simulink model "Demo_TollSystem_cs"  (R2014b)
settings: Solver=FixedStepDiscrete  StartTime=0.0  StopTime=13  FixedStep=1/20  RelTol=1e-3
PreLoadFcn:
  | mbxruntime.callbacks.PreLoadFcn(bdroot);
  | check_NUTS_defined
  | model_closed = 0;
  | assignin('base',['model_closed_' bdroot],false);
PostLoadFcn:
  | mbxruntime.callbacks.PostLoadFcn(bdroot);
InitFcn:
  | mbxruntime.callbacks.InitFcn(bdroot);
StartFcn:
  | mbxruntime.callbacks.StartFcn(bdroot);
  | 
  | open_system([bdroot '/Scope Plot']);
StopFcn:
  | mbxruntime.callbacks.StopFcn(bdroot);
model workspace: external: MAT-File .\Demo_TollSystem_cs_hws.mat (data not in the file)
undefined symbols (not defined in the file): Demo_TollSystem_cs_acfd828c7254e63e, Demo_TollSystem_cs_Mazda_RX8_1_Path_pathUniqueID
libraries: simulink x8, PreScanUsefulBlocks x4
(part 2 of 3)

== system Demo_TollSystem_cs/RFBeacon_3 ==
  Sensor : S-Function  FunctionName=sfun_Beacon  Parameters=sensorID, NrEntitiesOut, timestep  EnableBusSupport=off  mask(PreScan Source Block: RFBeacon I/O){sensorID=44, NrEntitiesOut=5, timestep=1/20}
      mask prompts: sensorID "Sensor ID"; NrEntitiesOut "User Specified: # of Visible OBUs"; timestep "MATLAB timestep:"
      mask help:
      | Using the Beacon and OBU (On-Board Unit) information between actors and infrastructure can be exchanged.
      |
      | The Beacon Receiver receives actor information and user-definable signals.
      |
      | For more information, please click Help.
      mask Help: eval('openHelp(486)')
      mask Display: image(imread('ico_Beacon_RF_24_gray.png'))
  RFBeacon_3 : Outport  Tag=outport/BeaconAndOBU/RFBeaconSensor  OutDataTypeStr=Bus: PRESCAN_BEACON_MESSAGE  PortDimensions=5  SampleTime=1/20
  wires:
  Sensor/1 -> RFBeacon_3/1

== system Demo_TollSystem_cs/RFBeacon_3Out ==
  RFBeacon_3Out : Inport  Tag=inport/BeaconAndOBU/RFBeaconSensor  OutDataTypeStr=Bus: PRESCAN_BEACONOBU_INPUT_DATA  PortDimensions=1  SampleTime=1/20  BusOutputAsStruct=on
  Actuator : S-Function  FunctionName=sfun_BeaconOBU_Input  Parameters=sensorID, timestep  EnableBusSupport=off  mask(PreScan Sink Block: RFBeacon I/O){sensorID=44, timestep=1/20}
      mask prompts: sensorID "Sensor ID"; timestep "MATLAB timestep:"
      mask help:
      | Using the Beacon and OBU (On-Board Unit) information between actors and infrastructure can be exchanged.
      |
      | The Beacon Transmitter contains the following, user-definable signals:
      |
      | - Beacon Type		[-]
      | - Spares (1:15)		[-]
      |
      | For more information, please click Help.
      mask Help: eval('openHelp(486)')
      mask Display: image(imread('ico_Beacon_RF_24_gray.png'))
  wires:
  RFBeacon_3Out/1 -> Actuator/1

== system Demo_TollSystem_cs/RFOBU_1 ==
  Sensor : S-Function  FunctionName=sfun_OBU  Parameters=sensorID, NrEntitiesOut, timestep  EnableBusSupport=off  mask(PreScan Source Block: RFOBU I/O){sensorID=17, NrEntitiesOut=2, timestep=1/20}
      mask prompts: sensorID "Sensor ID"; NrEntitiesOut "User Specified: # of Visible OBUs"; timestep "MATLAB timestep:"
      mask help:
      | Using the Beacon and OBU (On-Board Unit) information between actors and infrastructure can be exchanged.
      |
      | The OBU Receiver receives infrastructure information and user-definable signals.
      |
      | For more information, please click Help.
      mask Help: eval('openHelp(487)')
      mask Display: image(imread('ico_OBU_RF_24_gray.png'))
  RFOBU_1 : Outport  Tag=outport/BeaconAndOBU/RFOBU  OutDataTypeStr=Bus: PRESCAN_OBU_MESSAGE  PortDimensions=2  SampleTime=1/20
  wires:
  Sensor/1 -> RFOBU_1/1

== system Demo_TollSystem_cs/RFOBU_1Out ==
  RFOBU_1Out : Inport  Tag=inport/BeaconAndOBU/RFOBU  OutDataTypeStr=Bus: PRESCAN_BEACONOBU_INPUT_DATA  PortDimensions=1  SampleTime=1/20  BusOutputAsStruct=on
  Actuator : S-Function  FunctionName=sfun_BeaconOBU_Input  Parameters=sensorID, timestep  EnableBusSupport=off  mask(PreScan Sink Block: RFOBU I/O){sensorID=17, timestep=1/20}
      mask prompts: sensorID "Sensor ID"; timestep "MATLAB timestep:"
      mask help:
      | Using the Beacon and OBU (On-Board Unit) information between actors and infrastructure can be exchanged.
      |
      | The OBU Transmitter contains the following, user-definable signals:
      |
      | - Vehicle Type		[-]
      | - Spares (1:15)		[-]
      |
      | For more information, please click Help.
      mask Help: eval('openHelp(487)')
      mask Display: image(imread('ico_OBU_RF_24_gray.png'))
  wires:
  RFOBU_1Out/1 -> Actuator/1

== system Demo_TollSystem_cs/SELF_Mazda_RX8_1 ==
  Sensor : S-Function  FunctionName=sfun_SelfSensor  Parameters=UniqueID, TimeStep  EnableBusSupport=off  mask(PreScan Source Block: SELF){UniqueID=16, TimeStep=1/20}
      mask prompts: UniqueID "Auto-Assigned: Unique ID"; TimeStep "Auto-Assigned: Upload Period [s]"
      mask help:
      | The SELF port shows (state) information of the actor itself. The outputs are position in the experiment's axis system and the GPS coordinates, and the object's absolute velocity and compass heading.
      |
      | For more information, please click Help.
      mask Help: eval('openHelp(462)')
      mask Display: image(imread('GPS.png'))
  SELF_Mazda_RX8_1 : Outport  Tag=outport/SelfPort  OutDataTypeStr=Bus: PRESCAN_SELFSENSORDATA  PortDimensions=1  SampleTime=1/20
  wires:
  Sensor/1 -> SELF_Mazda_RX8_1/1

== system Demo_TollSystem_cs/STATE_Mazda_RX8_1_bus ==
  STATE_Mazda_RX8_1_bus : Inport  Tag=inport/StatePort  OutDataTypeStr=Bus: PRESCAN_STATEACTUATORDATA  PortDimensions=1  SampleTime=1/20  BusOutputAsStruct=on
  Actuator : S-Function  FunctionName=sfun_StateActuator  Parameters=UniqueID, TimeStep  EnableBusSupport=off  mask(PreScan Sink Block: State){UniqueID=16, TimeStep=1/20}
      mask prompts: UniqueID "Auto-Assigned: Unique ID"; TimeStep "Auto-Assigned: Upload Period [s]"
      mask help:
      | The Actor State contains a vector signal of size (9x1), containing the following signals:
      |
      | -  Position    	(x,y,z)             	[m]
      | -  Velocity    	(vx,vy,vz)         	[m/s]
      | -  Angles       	(Roll, Pitch, Yaw)	[rad]
      |
      | The Actor state is defined in the global axis system.
      | The state is superponed on the Initial position defined in the GUI.
      |
      | For more information, please click Help.
      mask Help: eval('openHelp(222)')
      mask Display: image(imread('State.png'))
  wires:
  STATE_Mazda_RX8_1_bus/1 -> Actuator/1

== system Demo_TollSystem_cs/ScenarioEngine ==
  Clock : Clock
  sfun_ScenarioEngine : S-Function  FunctionName=sfun_ScenarioEngine  Parameters=TimeStep  EnableBusSupport=off
  wires:
  Clock/1 -> sfun_ScenarioEngine/1

== system Demo_TollSystem_cs/Synchronizer ==
  Bus Selector1 : BusSelector  OutputSignals=FederateStopped
  Stop Simulation : Stop
  sfun_Synchronizer : S-Function  FunctionName=sfun_Synchronizer  Parameters=SampleTime  EnableBusSupport=off  mask(Legacy Function){SFunctionSpec=void prescan_synchronizer_outputFcn(void ** work1, PRESCAN_SYNCHRONIZEDATA y1[1]), SampleTime=TimeStep, ShowSpec=on}
      mask prompts: SampleTime "Sample time (-1 for inherited):"; ShowSpec "Display function specification"
      mask help:
      | This block allows you to call the legacy functions specified by the following Legacy Code Tool definition:
      | def.SFunctionName = 'sfun_Synchronizer';
      | def.OutputFcnSpec = 'void prescan_synchronizer_outputFcn(void ** work1, PRESCAN_SYNCHRONIZEDATA y1[1])';
      | def.StartFcnSpec = 'void prescan_synchronizer_startFcn(void ** work1)';
      | def.TerminateFcnSpec = 'void prescan_synchronizer_terminateFcn(void ** work1)';
      | def.HeaderFiles = {'prescan_synchronizer_data.h'};
      | def.HostLibFiles = {'sensorinterfaced.lib'};
      | def.IncPaths = {'src', 'C:\prescandev\vislibrary\vis\..\pimp\include\sensors\InterfaceRTW'};
      | def.SrcPaths = {'src'};
      | def.LibPaths = {'C:\\prescandev\\vislibrary_build\lib'};
      | def.SampleTime = 'parameterized';
      | def.Options.language = 'C';
      mask Help: <p>This block was generated automatically by the Legacy Code Tool. For detailed help on this tool, call<a href="matlab:legacy_code('help')"> legacy_code('help')</a>.</p>
      mask Callback ShowSpec:
      | if strcmp(get_param(gcbh, 'ShowSpec'), 'on')
      |   set_param(gcbh, 'MaskDisplay', sprintf('fprintf(''%s'');', get_param(gcbh, 'SFunctionSpec')));
      | else
      |   set_param(gcbh, 'MaskDisplay', sprintf('fprintf(''%s'');', get_param(gcbh, 'FunctionName')));
      | end
      mask Display: fprintf('void prescan_synchronizer_outputFcn(void ** work1, PRESCAN_SYNCHRONIZEDATA y1[1])');
  wires:
  Bus Selector1/1 -> Stop Simulation/1  "<FederateStopped>"
  sfun_Synchronizer/1 -> Bus Selector1/1

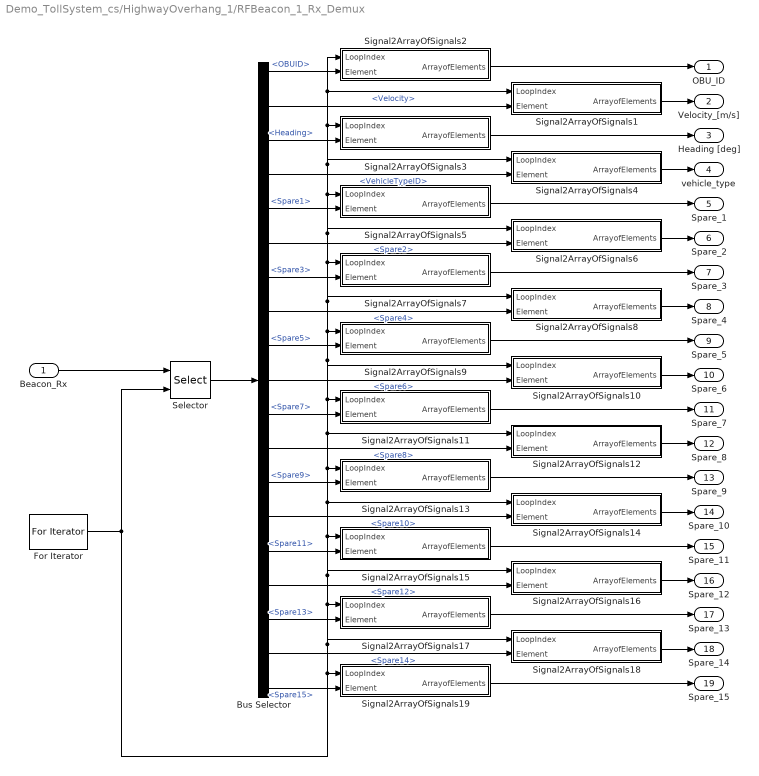
== system Demo_TollSystem_cs/HighwayOverhang_1/RFBeacon_1_Rx_Demux ==
  Beacon_Rx : Inport
  Bus Selector : BusSelector  OutputSignals=DATA.OBUID,DATA.Velocity,DATA.Heading,DATA.VehicleTypeID,DATA.Spare1,DATA.Spare2,DATA.Spare3,DATA.Spare4,DATA.Spare5,DATA.Spare6,DATA.Spare7,DATA.Spare8,DATA.Spare9,DATA.Spare10,DATA.Spare11,DATA.Spare12,DATA.Spare13,DATA.Spare14,DATA.Spare15
  For Iterator : ForIterator  ResetStates=reset  IterationLimit=detectableObjects
  Selector : Selector  InputPortWidth=detectableObjects  IndexOptions=Index vector (port)  Indices=[1 3]
  Signal2ArrayOfSignals1 : Subsystem  mask{VECTORLENGTH=detectableObjects}
      mask prompts: VECTORLENGTH "Length of vector"
  Signal2ArrayOfSignals10 : Subsystem  mask{VECTORLENGTH=detectableObjects}
      mask prompts: VECTORLENGTH "Length of vector"
  Signal2ArrayOfSignals11 : Subsystem  mask{VECTORLENGTH=detectableObjects}
      mask prompts: VECTORLENGTH "Length of vector"
  Signal2ArrayOfSignals12 : Subsystem  mask{VECTORLENGTH=detectableObjects}
      mask prompts: VECTORLENGTH "Length of vector"
  Signal2ArrayOfSignals13 : Subsystem  mask{VECTORLENGTH=detectableObjects}
      mask prompts: VECTORLENGTH "Length of vector"
  Signal2ArrayOfSignals14 : Subsystem  mask{VECTORLENGTH=detectableObjects}
      mask prompts: VECTORLENGTH "Length of vector"
  Signal2ArrayOfSignals15 : Subsystem  mask{VECTORLENGTH=detectableObjects}
      mask prompts: VECTORLENGTH "Length of vector"
  Signal2ArrayOfSignals16 : Subsystem  mask{VECTORLENGTH=detectableObjects}
      mask prompts: VECTORLENGTH "Length of vector"
  Signal2ArrayOfSignals17 : Subsystem  mask{VECTORLENGTH=detectableObjects}
      mask prompts: VECTORLENGTH "Length of vector"
  Signal2ArrayOfSignals18 : Subsystem  mask{VECTORLENGTH=detectableObjects}
      mask prompts: VECTORLENGTH "Length of vector"
  Signal2ArrayOfSignals19 : Subsystem  mask{VECTORLENGTH=detectableObjects}
      mask prompts: VECTORLENGTH "Length of vector"
  Signal2ArrayOfSignals2 : Subsystem  mask{VECTORLENGTH=detectableObjects}
      mask prompts: VECTORLENGTH "Length of vector"
  Signal2ArrayOfSignals3 : Subsystem  mask{VECTORLENGTH=detectableObjects}
      mask prompts: VECTORLENGTH "Length of vector"
  Signal2ArrayOfSignals4 : Subsystem  mask{VECTORLENGTH=detectableObjects}
      mask prompts: VECTORLENGTH "Length of vector"
  Signal2ArrayOfSignals5 : Subsystem  mask{VECTORLENGTH=detectableObjects}
      mask prompts: VECTORLENGTH "Length of vector"
  Signal2ArrayOfSignals6 : Subsystem  mask{VECTORLENGTH=detectableObjects}
      mask prompts: VECTORLENGTH "Length of vector"
  Signal2ArrayOfSignals7 : Subsystem  mask{VECTORLENGTH=detectableObjects}
      mask prompts: VECTORLENGTH "Length of vector"
  Signal2ArrayOfSignals8 : Subsystem  mask{VECTORLENGTH=detectableObjects}
      mask prompts: VECTORLENGTH "Length of vector"
  Signal2ArrayOfSignals9 : Subsystem  mask{VECTORLENGTH=detectableObjects}
      mask prompts: VECTORLENGTH "Length of vector"
  OBU_ID : Outport
  Velocity_[m/s] : Outport  Port=2
  Heading [deg] : Outport  Port=3
  vehicle_type : Outport  Port=4
  Spare_1 : Outport  Port=5
  Spare_2 : Outport  Port=6
  Spare_3 : Outport  Port=7
  Spare_4 : Outport  Port=8
  Spare_5 : Outport  Port=9
  Spare_6 : Outport  Port=10
  Spare_7 : Outport  Port=11
  Spare_8 : Outport  Port=12
  Spare_9 : Outport  Port=13
  Spare_10 : Outport  Port=14
  Spare_11 : Outport  Port=15
  Spare_12 : Outport  Port=16
  Spare_13 : Outport  Port=17
  Spare_14 : Outport  Port=18
  Spare_15 : Outport  Port=19
  wires:
  Beacon_Rx/1 -> Selector/1
  For Iterator/1 -> Selector/2, Signal2ArrayOfSignals19/1(LoopIndex), Signal2ArrayOfSignals17/1(LoopIndex), Signal2ArrayOfSignals15/1(LoopIndex), Signal2ArrayOfSignals13/1(LoopIndex), Signal2ArrayOfSignals11/1(LoopIndex), Signal2ArrayOfSignals9/1(LoopIndex), Signal2ArrayOfSignals7/1(LoopIndex), Signal2ArrayOfSignals5/1(LoopIndex), Signal2ArrayOfSignals3/1(LoopIndex), Signal2ArrayOfSignals2/1(LoopIndex), Signal2ArrayOfSignals1/1(LoopIndex), Signal2ArrayOfSignals4/1(LoopIndex), Signal2ArrayOfSignals6/1(LoopIndex), Signal2ArrayOfSignals8/1(LoopIndex), Signal2ArrayOfSignals10/1(LoopIndex), Signal2ArrayOfSignals12/1(LoopIndex), Signal2ArrayOfSignals14/1(LoopIndex), Signal2ArrayOfSignals16/1(LoopIndex), Signal2ArrayOfSignals18/1(LoopIndex)
  Selector/1 -> Bus Selector/1
  Bus Selector/1 -> Signal2ArrayOfSignals2/2(Element)  "<OBUID>"
  Signal2ArrayOfSignals2/1(ArrayofElements) -> OBU_ID/1
  Bus Selector/2 -> Signal2ArrayOfSignals1/2(Element)  "<Velocity>"
  Signal2ArrayOfSignals1/1(ArrayofElements) -> Velocity_[m/s]/1
  Bus Selector/3 -> Signal2ArrayOfSignals3/2(Element)  "<Heading>"
  Signal2ArrayOfSignals3/1(ArrayofElements) -> Heading [deg]/1
  Bus Selector/4 -> Signal2ArrayOfSignals4/2(Element)  "<VehicleTypeID>"
  Signal2ArrayOfSignals4/1(ArrayofElements) -> vehicle_type/1
  Bus Selector/5 -> Signal2ArrayOfSignals5/2(Element)  "<Spare1>"
  Signal2ArrayOfSignals5/1(ArrayofElements) -> Spare_1/1
  Bus Selector/6 -> Signal2ArrayOfSignals6/2(Element)  "<Spare2>"
  Signal2ArrayOfSignals6/1(ArrayofElements) -> Spare_2/1
  Bus Selector/7 -> Signal2ArrayOfSignals7/2(Element)  "<Spare3>"
  Signal2ArrayOfSignals7/1(ArrayofElements) -> Spare_3/1
  Bus Selector/8 -> Signal2ArrayOfSignals8/2(Element)  "<Spare4>"
  Signal2ArrayOfSignals8/1(ArrayofElements) -> Spare_4/1
  Bus Selector/9 -> Signal2ArrayOfSignals9/2(Element)  "<Spare5>"
  Bus Selector/10 -> Signal2ArrayOfSignals10/2(Element)  "<Spare6>"
  Bus Selector/11 -> Signal2ArrayOfSignals11/2(Element)  "<Spare7>"
  Bus Selector/12 -> Signal2ArrayOfSignals12/2(Element)  "<Spare8>"
  Signal2ArrayOfSignals9/1(ArrayofElements) -> Spare_5/1
  Signal2ArrayOfSignals10/1(ArrayofElements) -> Spare_6/1
  Signal2ArrayOfSignals11/1(ArrayofElements) -> Spare_7/1
  Signal2ArrayOfSignals12/1(ArrayofElements) -> Spare_8/1
  Bus Selector/13 -> Signal2ArrayOfSignals13/2(Element)  "<Spare9>"
  Bus Selector/14 -> Signal2ArrayOfSignals14/2(Element)  "<Spare10>"
  Signal2ArrayOfSignals13/1(ArrayofElements) -> Spare_9/1
  Signal2ArrayOfSignals14/1(ArrayofElements) -> Spare_10/1
  Bus Selector/15 -> Signal2ArrayOfSignals15/2(Element)  "<Spare11>"
  Signal2ArrayOfSignals15/1(ArrayofElements) -> Spare_11/1
  Bus Selector/16 -> Signal2ArrayOfSignals16/2(Element)  "<Spare12>"
  Signal2ArrayOfSignals16/1(ArrayofElements) -> Spare_12/1
  Bus Selector/17 -> Signal2ArrayOfSignals17/2(Element)  "<Spare13>"
  Signal2ArrayOfSignals17/1(ArrayofElements) -> Spare_13/1
  Bus Selector/18 -> Signal2ArrayOfSignals18/2(Element)  "<Spare14>"
  Signal2ArrayOfSignals18/1(ArrayofElements) -> Spare_14/1
  Bus Selector/19 -> Signal2ArrayOfSignals19/2(Element)  "<Spare15>"
  Signal2ArrayOfSignals19/1(ArrayofElements) -> Spare_15/1

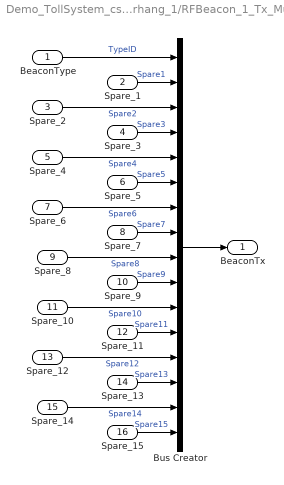
== system Demo_TollSystem_cs/HighwayOverhang_1/RFBeacon_1_Tx_Mux ==
  BeaconType : Inport
  Spare_1 : Inport  Port=2
  Spare_2 : Inport  Port=3
  Spare_3 : Inport  Port=4
  Spare_4 : Inport  Port=5
  Spare_5 : Inport  Port=6
  Spare_6 : Inport  Port=7
  Spare_7 : Inport  Port=8
  Spare_8 : Inport  Port=9
  Spare_9 : Inport  Port=10
  Spare_10 : Inport  Port=11
  Spare_11 : Inport  Port=12
  Spare_12 : Inport  Port=13
  Spare_13 : Inport  Port=14
  Spare_14 : Inport  Port=15
  Spare_15 : Inport  Port=16
  Bus Creator : BusCreator  Inputs=16  OutDataTypeStr=Bus: PRESCAN_BEACONOBU_INPUT_DATA
  BeaconTx : Outport
  wires:
  Spare_11/1 -> Bus Creator/12  "Spare11"
  Spare_12/1 -> Bus Creator/13  "Spare12"
  Spare_13/1 -> Bus Creator/14  "Spare13"
  Spare_14/1 -> Bus Creator/15  "Spare14"
  Spare_15/1 -> Bus Creator/16  "Spare15"
  Spare_1/1 -> Bus Creator/2  "Spare1"
  Spare_2/1 -> Bus Creator/3  "Spare2"
  Spare_3/1 -> Bus Creator/4  "Spare3"
  Spare_4/1 -> Bus Creator/5  "Spare4"
  Spare_5/1 -> Bus Creator/6  "Spare5"
  Spare_6/1 -> Bus Creator/7  "Spare6"
  Spare_7/1 -> Bus Creator/8  "Spare7"
  Spare_8/1 -> Bus Creator/9  "Spare8"
  Spare_9/1 -> Bus Creator/10  "Spare9"
  Spare_10/1 -> Bus Creator/11  "Spare10"
  Bus Creator/1 -> BeaconTx/1
  BeaconType/1 -> Bus Creator/1  "TypeID"

== system Demo_TollSystem_cs/HighwayOverhang_1/threshold check ==
  Lat : Inport
  Lon : Inport  Port=2
  Pos Lat : Inport  Port=3
  Pos Lon : Inport  Port=4
  Abs : Abs
  Abs1 : Abs
  Accuracy : Constant  Value=1e-5
  Compare To Zero : simulink/Logic and Bit Operations/Compare To Zero  relop=~=  OutDataTypeStr=uint8  ZeroCross=off
  Compare To Zero1 : simulink/Logic and Bit Operations/Compare To Zero  relop=~=  OutDataTypeStr=uint8  ZeroCross=off
  Logical Operator : Logic  Inputs=3  AllPortsSameDT=off  OutDataTypeStr=boolean
  Logical Operator1 : Logic  Operator=OR  AllPortsSameDT=off  OutDataTypeStr=boolean
  Relational Operator : RelationalOperator  Operator=>  OutDataTypeStr=boolean
  Relational Operator1 : RelationalOperator  Operator=>  OutDataTypeStr=boolean
  Sum : Sum  Inputs=|+-
  Sum1 : Sum  Inputs=|+-
  Out : Outport
  wires:
  Pos Lat/1 -> Sum/2
  Lat/1 -> Sum/1, Compare To Zero/1
  Sum/1 -> Abs/1
  Pos Lon/1 -> Sum1/2
  Lon/1 -> Sum1/1, Compare To Zero1/1
  Sum1/1 -> Abs1/1
  Relational Operator/1 -> Logical Operator1/1
  Logical Operator/1 -> Out/1
  Abs/1 -> Relational Operator/1
  Accuracy/1 -> Relational Operator/2, Relational Operator1/2
  Abs1/1 -> Relational Operator1/1
  Compare To Zero/1 -> Logical Operator/1
  Compare To Zero1/1 -> Logical Operator1/2
  Relational Operator1/1 -> Logical Operator/3
  Logical Operator1/1 -> Logical Operator/2

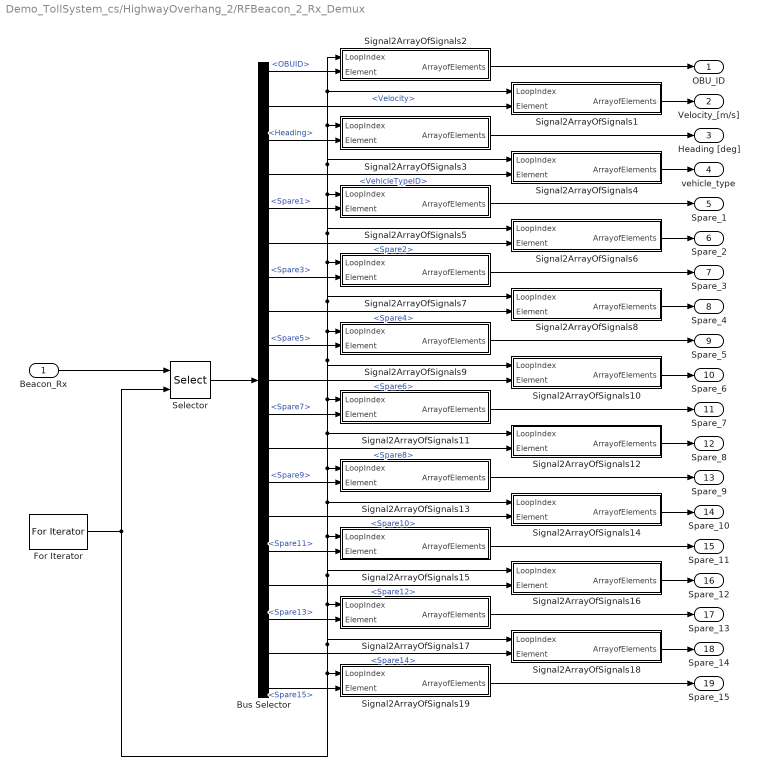
== system Demo_TollSystem_cs/HighwayOverhang_2/RFBeacon_2_Rx_Demux ==
  Beacon_Rx : Inport
  Bus Selector : BusSelector  OutputSignals=DATA.OBUID,DATA.Velocity,DATA.Heading,DATA.VehicleTypeID,DATA.Spare1,DATA.Spare2,DATA.Spare3,DATA.Spare4,DATA.Spare5,DATA.Spare6,DATA.Spare7,DATA.Spare8,DATA.Spare9,DATA.Spare10,DATA.Spare11,DATA.Spare12,DATA.Spare13,DATA.Spare14,DATA.Spare15
  For Iterator : ForIterator  ResetStates=reset  IterationLimit=detectableObjects
  Selector : Selector  InputPortWidth=detectableObjects  IndexOptions=Index vector (port)  Indices=[1 3]
  Signal2ArrayOfSignals1 : Subsystem  mask{VECTORLENGTH=detectableObjects}
      mask prompts: VECTORLENGTH "Length of vector"
  Signal2ArrayOfSignals10 : Subsystem  mask{VECTORLENGTH=detectableObjects}
      mask prompts: VECTORLENGTH "Length of vector"
  Signal2ArrayOfSignals11 : Subsystem  mask{VECTORLENGTH=detectableObjects}
      mask prompts: VECTORLENGTH "Length of vector"
  Signal2ArrayOfSignals12 : Subsystem  mask{VECTORLENGTH=detectableObjects}
      mask prompts: VECTORLENGTH "Length of vector"
  Signal2ArrayOfSignals13 : Subsystem  mask{VECTORLENGTH=detectableObjects}
      mask prompts: VECTORLENGTH "Length of vector"
  Signal2ArrayOfSignals14 : Subsystem  mask{VECTORLENGTH=detectableObjects}
      mask prompts: VECTORLENGTH "Length of vector"
  Signal2ArrayOfSignals15 : Subsystem  mask{VECTORLENGTH=detectableObjects}
      mask prompts: VECTORLENGTH "Length of vector"
  Signal2ArrayOfSignals16 : Subsystem  mask{VECTORLENGTH=detectableObjects}
      mask prompts: VECTORLENGTH "Length of vector"
  Signal2ArrayOfSignals17 : Subsystem  mask{VECTORLENGTH=detectableObjects}
      mask prompts: VECTORLENGTH "Length of vector"
  Signal2ArrayOfSignals18 : Subsystem  mask{VECTORLENGTH=detectableObjects}
      mask prompts: VECTORLENGTH "Length of vector"
  Signal2ArrayOfSignals19 : Subsystem  mask{VECTORLENGTH=detectableObjects}
      mask prompts: VECTORLENGTH "Length of vector"
  Signal2ArrayOfSignals2 : Subsystem  mask{VECTORLENGTH=detectableObjects}
      mask prompts: VECTORLENGTH "Length of vector"
  Signal2ArrayOfSignals3 : Subsystem  mask{VECTORLENGTH=detectableObjects}
      mask prompts: VECTORLENGTH "Length of vector"
  Signal2ArrayOfSignals4 : Subsystem  mask{VECTORLENGTH=detectableObjects}
      mask prompts: VECTORLENGTH "Length of vector"
  Signal2ArrayOfSignals5 : Subsystem  mask{VECTORLENGTH=detectableObjects}
      mask prompts: VECTORLENGTH "Length of vector"
  Signal2ArrayOfSignals6 : Subsystem  mask{VECTORLENGTH=detectableObjects}
      mask prompts: VECTORLENGTH "Length of vector"
  Signal2ArrayOfSignals7 : Subsystem  mask{VECTORLENGTH=detectableObjects}
      mask prompts: VECTORLENGTH "Length of vector"
  Signal2ArrayOfSignals8 : Subsystem  mask{VECTORLENGTH=detectableObjects}
      mask prompts: VECTORLENGTH "Length of vector"
  Signal2ArrayOfSignals9 : Subsystem  mask{VECTORLENGTH=detectableObjects}
      mask prompts: VECTORLENGTH "Length of vector"
  OBU_ID : Outport
  Velocity_[m/s] : Outport  Port=2
  Heading [deg] : Outport  Port=3
  vehicle_type : Outport  Port=4
  Spare_1 : Outport  Port=5
  Spare_2 : Outport  Port=6
  Spare_3 : Outport  Port=7
  Spare_4 : Outport  Port=8
  Spare_5 : Outport  Port=9
  Spare_6 : Outport  Port=10
  Spare_7 : Outport  Port=11
  Spare_8 : Outport  Port=12
  Spare_9 : Outport  Port=13
  Spare_10 : Outport  Port=14
  Spare_11 : Outport  Port=15
  Spare_12 : Outport  Port=16
  Spare_13 : Outport  Port=17
  Spare_14 : Outport  Port=18
  Spare_15 : Outport  Port=19
  wires:
  Beacon_Rx/1 -> Selector/1
  For Iterator/1 -> Selector/2, Signal2ArrayOfSignals19/1(LoopIndex), Signal2ArrayOfSignals17/1(LoopIndex), Signal2ArrayOfSignals15/1(LoopIndex), Signal2ArrayOfSignals13/1(LoopIndex), Signal2ArrayOfSignals11/1(LoopIndex), Signal2ArrayOfSignals9/1(LoopIndex), Signal2ArrayOfSignals7/1(LoopIndex), Signal2ArrayOfSignals5/1(LoopIndex), Signal2ArrayOfSignals3/1(LoopIndex), Signal2ArrayOfSignals2/1(LoopIndex), Signal2ArrayOfSignals1/1(LoopIndex), Signal2ArrayOfSignals4/1(LoopIndex), Signal2ArrayOfSignals6/1(LoopIndex), Signal2ArrayOfSignals8/1(LoopIndex), Signal2ArrayOfSignals10/1(LoopIndex), Signal2ArrayOfSignals12/1(LoopIndex), Signal2ArrayOfSignals14/1(LoopIndex), Signal2ArrayOfSignals16/1(LoopIndex), Signal2ArrayOfSignals18/1(LoopIndex)
  Selector/1 -> Bus Selector/1
  Bus Selector/1 -> Signal2ArrayOfSignals2/2(Element)  "<OBUID>"
  Signal2ArrayOfSignals2/1(ArrayofElements) -> OBU_ID/1
  Bus Selector/2 -> Signal2ArrayOfSignals1/2(Element)  "<Velocity>"
  Signal2ArrayOfSignals1/1(ArrayofElements) -> Velocity_[m/s]/1
  Bus Selector/3 -> Signal2ArrayOfSignals3/2(Element)  "<Heading>"
  Signal2ArrayOfSignals3/1(ArrayofElements) -> Heading [deg]/1
  Bus Selector/4 -> Signal2ArrayOfSignals4/2(Element)  "<VehicleTypeID>"
  Signal2ArrayOfSignals4/1(ArrayofElements) -> vehicle_type/1
  Bus Selector/5 -> Signal2ArrayOfSignals5/2(Element)  "<Spare1>"
  Signal2ArrayOfSignals5/1(ArrayofElements) -> Spare_1/1
  Bus Selector/6 -> Signal2ArrayOfSignals6/2(Element)  "<Spare2>"
  Signal2ArrayOfSignals6/1(ArrayofElements) -> Spare_2/1
  Bus Selector/7 -> Signal2ArrayOfSignals7/2(Element)  "<Spare3>"
  Signal2ArrayOfSignals7/1(ArrayofElements) -> Spare_3/1
  Bus Selector/8 -> Signal2ArrayOfSignals8/2(Element)  "<Spare4>"
  Signal2ArrayOfSignals8/1(ArrayofElements) -> Spare_4/1
  Bus Selector/9 -> Signal2ArrayOfSignals9/2(Element)  "<Spare5>"
  Bus Selector/10 -> Signal2ArrayOfSignals10/2(Element)  "<Spare6>"
  Bus Selector/11 -> Signal2ArrayOfSignals11/2(Element)  "<Spare7>"
  Bus Selector/12 -> Signal2ArrayOfSignals12/2(Element)  "<Spare8>"
  Signal2ArrayOfSignals9/1(ArrayofElements) -> Spare_5/1
  Signal2ArrayOfSignals10/1(ArrayofElements) -> Spare_6/1
  Signal2ArrayOfSignals11/1(ArrayofElements) -> Spare_7/1
  Signal2ArrayOfSignals12/1(ArrayofElements) -> Spare_8/1
  Bus Selector/13 -> Signal2ArrayOfSignals13/2(Element)  "<Spare9>"
  Bus Selector/14 -> Signal2ArrayOfSignals14/2(Element)  "<Spare10>"
  Signal2ArrayOfSignals13/1(ArrayofElements) -> Spare_9/1
  Signal2ArrayOfSignals14/1(ArrayofElements) -> Spare_10/1
  Bus Selector/15 -> Signal2ArrayOfSignals15/2(Element)  "<Spare11>"
  Signal2ArrayOfSignals15/1(ArrayofElements) -> Spare_11/1
  Bus Selector/16 -> Signal2ArrayOfSignals16/2(Element)  "<Spare12>"
  Signal2ArrayOfSignals16/1(ArrayofElements) -> Spare_12/1
  Bus Selector/17 -> Signal2ArrayOfSignals17/2(Element)  "<Spare13>"
  Signal2ArrayOfSignals17/1(ArrayofElements) -> Spare_13/1
  Bus Selector/18 -> Signal2ArrayOfSignals18/2(Element)  "<Spare14>"
  Signal2ArrayOfSignals18/1(ArrayofElements) -> Spare_14/1
  Bus Selector/19 -> Signal2ArrayOfSignals19/2(Element)  "<Spare15>"
  Signal2ArrayOfSignals19/1(ArrayofElements) -> Spare_15/1

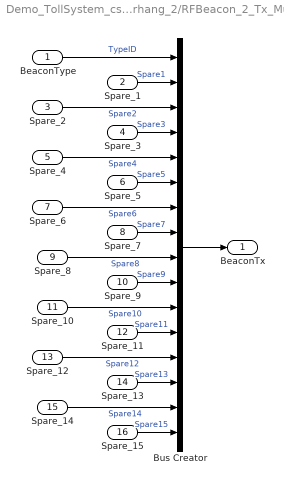
== system Demo_TollSystem_cs/HighwayOverhang_2/RFBeacon_2_Tx_Mux ==
  BeaconType : Inport
  Spare_1 : Inport  Port=2
  Spare_2 : Inport  Port=3
  Spare_3 : Inport  Port=4
  Spare_4 : Inport  Port=5
  Spare_5 : Inport  Port=6
  Spare_6 : Inport  Port=7
  Spare_7 : Inport  Port=8
  Spare_8 : Inport  Port=9
  Spare_9 : Inport  Port=10
  Spare_10 : Inport  Port=11
  Spare_11 : Inport  Port=12
  Spare_12 : Inport  Port=13
  Spare_13 : Inport  Port=14
  Spare_14 : Inport  Port=15
  Spare_15 : Inport  Port=16
  Bus Creator : BusCreator  Inputs=16  OutDataTypeStr=Bus: PRESCAN_BEACONOBU_INPUT_DATA
  BeaconTx : Outport
  wires:
  Spare_11/1 -> Bus Creator/12  "Spare11"
  Spare_12/1 -> Bus Creator/13  "Spare12"
  Spare_13/1 -> Bus Creator/14  "Spare13"
  Spare_14/1 -> Bus Creator/15  "Spare14"
  Spare_15/1 -> Bus Creator/16  "Spare15"
  Spare_1/1 -> Bus Creator/2  "Spare1"
  Spare_2/1 -> Bus Creator/3  "Spare2"
  Spare_3/1 -> Bus Creator/4  "Spare3"
  Spare_4/1 -> Bus Creator/5  "Spare4"
  Spare_5/1 -> Bus Creator/6  "Spare5"
  Spare_6/1 -> Bus Creator/7  "Spare6"
  Spare_7/1 -> Bus Creator/8  "Spare7"
  Spare_8/1 -> Bus Creator/9  "Spare8"
  Spare_9/1 -> Bus Creator/10  "Spare9"
  Spare_10/1 -> Bus Creator/11  "Spare10"
  Bus Creator/1 -> BeaconTx/1
  BeaconType/1 -> Bus Creator/1  "TypeID"

== system Demo_TollSystem_cs/HighwayOverhang_2/threshold check ==
  Lat : Inport
  Lon : Inport  Port=2
  Pos Lat : Inport  Port=3
  Pos Lon : Inport  Port=4
  Abs : Abs
  Abs1 : Abs
  Accuracy : Constant  Value=1e-5
  Compare To Zero : simulink/Logic and Bit Operations/Compare To Zero  relop=~=  OutDataTypeStr=uint8  ZeroCross=off
  Compare To Zero1 : simulink/Logic and Bit Operations/Compare To Zero  relop=~=  OutDataTypeStr=uint8  ZeroCross=off
  Logical Operator : Logic  Inputs=3  AllPortsSameDT=off  OutDataTypeStr=float('double')
  Logical Operator1 : Logic  Operator=OR  AllPortsSameDT=off  OutDataTypeStr=boolean
  Relational Operator : RelationalOperator  Operator=>  OutDataTypeStr=boolean
  Relational Operator1 : RelationalOperator  Operator=>  OutDataTypeStr=boolean
  Sum : Sum  Inputs=|+-
  Sum1 : Sum  Inputs=|+-
  Out : Outport
  wires:
  Pos Lat/1 -> Sum/2
  Lat/1 -> Sum/1, Compare To Zero/1
  Sum/1 -> Abs/1
  Pos Lon/1 -> Sum1/2
  Lon/1 -> Sum1/1, Compare To Zero1/1
  Sum1/1 -> Abs1/1
  Relational Operator/1 -> Logical Operator1/1
  Logical Operator/1 -> Out/1
  Abs/1 -> Relational Operator/1
  Accuracy/1 -> Relational Operator/2, Relational Operator1/2
  Abs1/1 -> Relational Operator1/1
  Compare To Zero/1 -> Logical Operator/1
  Compare To Zero1/1 -> Logical Operator1/2
  Relational Operator1/1 -> Logical Operator/3
  Logical Operator1/1 -> Logical Operator/2

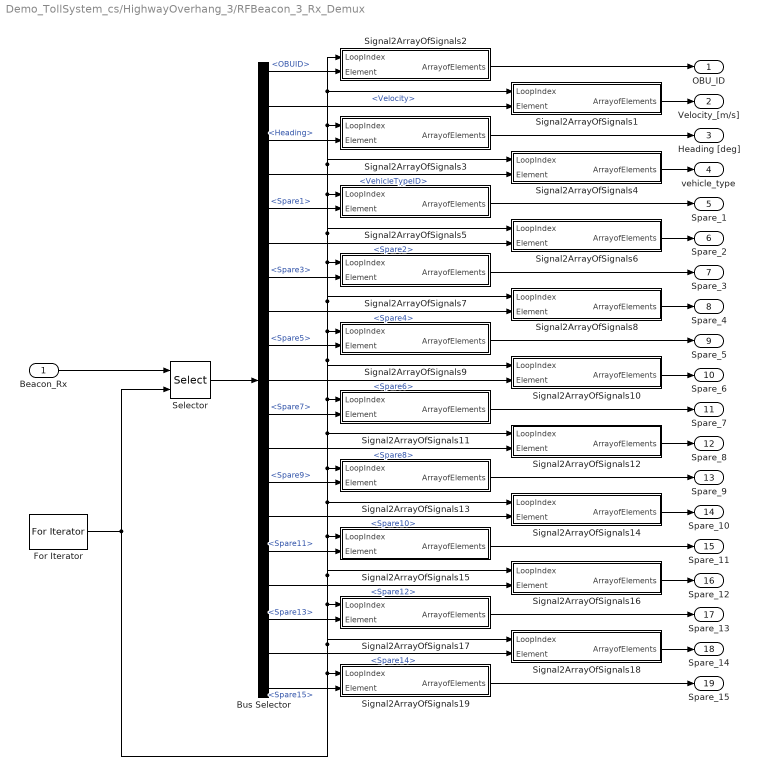
== system Demo_TollSystem_cs/HighwayOverhang_3/RFBeacon_3_Rx_Demux ==
  Beacon_Rx : Inport
  Bus Selector : BusSelector  OutputSignals=DATA.OBUID,DATA.Velocity,DATA.Heading,DATA.VehicleTypeID,DATA.Spare1,DATA.Spare2,DATA.Spare3,DATA.Spare4,DATA.Spare5,DATA.Spare6,DATA.Spare7,DATA.Spare8,DATA.Spare9,DATA.Spare10,DATA.Spare11,DATA.Spare12,DATA.Spare13,DATA.Spare14,DATA.Spare15
  For Iterator : ForIterator  ResetStates=reset  IterationLimit=detectableObjects
  Selector : Selector  InputPortWidth=detectableObjects  IndexOptions=Index vector (port)  Indices=[1 3]
  Signal2ArrayOfSignals1 : Subsystem  mask{VECTORLENGTH=detectableObjects}
      mask prompts: VECTORLENGTH "Length of vector"
  Signal2ArrayOfSignals10 : Subsystem  mask{VECTORLENGTH=detectableObjects}
      mask prompts: VECTORLENGTH "Length of vector"
  Signal2ArrayOfSignals11 : Subsystem  mask{VECTORLENGTH=detectableObjects}
      mask prompts: VECTORLENGTH "Length of vector"
  Signal2ArrayOfSignals12 : Subsystem  mask{VECTORLENGTH=detectableObjects}
      mask prompts: VECTORLENGTH "Length of vector"
  Signal2ArrayOfSignals13 : Subsystem  mask{VECTORLENGTH=detectableObjects}
      mask prompts: VECTORLENGTH "Length of vector"
  Signal2ArrayOfSignals14 : Subsystem  mask{VECTORLENGTH=detectableObjects}
      mask prompts: VECTORLENGTH "Length of vector"
  Signal2ArrayOfSignals15 : Subsystem  mask{VECTORLENGTH=detectableObjects}
      mask prompts: VECTORLENGTH "Length of vector"
  Signal2ArrayOfSignals16 : Subsystem  mask{VECTORLENGTH=detectableObjects}
      mask prompts: VECTORLENGTH "Length of vector"
  Signal2ArrayOfSignals17 : Subsystem  mask{VECTORLENGTH=detectableObjects}
      mask prompts: VECTORLENGTH "Length of vector"
  Signal2ArrayOfSignals18 : Subsystem  mask{VECTORLENGTH=detectableObjects}
      mask prompts: VECTORLENGTH "Length of vector"
  Signal2ArrayOfSignals19 : Subsystem  mask{VECTORLENGTH=detectableObjects}
      mask prompts: VECTORLENGTH "Length of vector"
  Signal2ArrayOfSignals2 : Subsystem  mask{VECTORLENGTH=detectableObjects}
      mask prompts: VECTORLENGTH "Length of vector"
  Signal2ArrayOfSignals3 : Subsystem  mask{VECTORLENGTH=detectableObjects}
      mask prompts: VECTORLENGTH "Length of vector"
  Signal2ArrayOfSignals4 : Subsystem  mask{VECTORLENGTH=detectableObjects}
      mask prompts: VECTORLENGTH "Length of vector"
  Signal2ArrayOfSignals5 : Subsystem  mask{VECTORLENGTH=detectableObjects}
      mask prompts: VECTORLENGTH "Length of vector"
  Signal2ArrayOfSignals6 : Subsystem  mask{VECTORLENGTH=detectableObjects}
      mask prompts: VECTORLENGTH "Length of vector"
  Signal2ArrayOfSignals7 : Subsystem  mask{VECTORLENGTH=detectableObjects}
      mask prompts: VECTORLENGTH "Length of vector"
  Signal2ArrayOfSignals8 : Subsystem  mask{VECTORLENGTH=detectableObjects}
      mask prompts: VECTORLENGTH "Length of vector"
  Signal2ArrayOfSignals9 : Subsystem  mask{VECTORLENGTH=detectableObjects}
      mask prompts: VECTORLENGTH "Length of vector"
  OBU_ID : Outport
  Velocity_[m/s] : Outport  Port=2
  Heading [deg] : Outport  Port=3
  vehicle_type : Outport  Port=4
  Spare_1 : Outport  Port=5
  Spare_2 : Outport  Port=6
  Spare_3 : Outport  Port=7
  Spare_4 : Outport  Port=8
  Spare_5 : Outport  Port=9
  Spare_6 : Outport  Port=10
  Spare_7 : Outport  Port=11
  Spare_8 : Outport  Port=12
  Spare_9 : Outport  Port=13
  Spare_10 : Outport  Port=14
  Spare_11 : Outport  Port=15
  Spare_12 : Outport  Port=16
  Spare_13 : Outport  Port=17
  Spare_14 : Outport  Port=18
  Spare_15 : Outport  Port=19
  wires:
  Beacon_Rx/1 -> Selector/1
  For Iterator/1 -> Selector/2, Signal2ArrayOfSignals19/1(LoopIndex), Signal2ArrayOfSignals17/1(LoopIndex), Signal2ArrayOfSignals15/1(LoopIndex), Signal2ArrayOfSignals13/1(LoopIndex), Signal2ArrayOfSignals11/1(LoopIndex), Signal2ArrayOfSignals9/1(LoopIndex), Signal2ArrayOfSignals7/1(LoopIndex), Signal2ArrayOfSignals5/1(LoopIndex), Signal2ArrayOfSignals3/1(LoopIndex), Signal2ArrayOfSignals2/1(LoopIndex), Signal2ArrayOfSignals1/1(LoopIndex), Signal2ArrayOfSignals4/1(LoopIndex), Signal2ArrayOfSignals6/1(LoopIndex), Signal2ArrayOfSignals8/1(LoopIndex), Signal2ArrayOfSignals10/1(LoopIndex), Signal2ArrayOfSignals12/1(LoopIndex), Signal2ArrayOfSignals14/1(LoopIndex), Signal2ArrayOfSignals16/1(LoopIndex), Signal2ArrayOfSignals18/1(LoopIndex)
  Selector/1 -> Bus Selector/1
  Bus Selector/1 -> Signal2ArrayOfSignals2/2(Element)  "<OBUID>"
  Signal2ArrayOfSignals2/1(ArrayofElements) -> OBU_ID/1
  Bus Selector/2 -> Signal2ArrayOfSignals1/2(Element)  "<Velocity>"
  Signal2ArrayOfSignals1/1(ArrayofElements) -> Velocity_[m/s]/1
  Bus Selector/3 -> Signal2ArrayOfSignals3/2(Element)  "<Heading>"
  Signal2ArrayOfSignals3/1(ArrayofElements) -> Heading [deg]/1
  Bus Selector/4 -> Signal2ArrayOfSignals4/2(Element)  "<VehicleTypeID>"
  Signal2ArrayOfSignals4/1(ArrayofElements) -> vehicle_type/1
  Bus Selector/5 -> Signal2ArrayOfSignals5/2(Element)  "<Spare1>"
  Signal2ArrayOfSignals5/1(ArrayofElements) -> Spare_1/1
  Bus Selector/6 -> Signal2ArrayOfSignals6/2(Element)  "<Spare2>"
  Signal2ArrayOfSignals6/1(ArrayofElements) -> Spare_2/1
  Bus Selector/7 -> Signal2ArrayOfSignals7/2(Element)  "<Spare3>"
  Signal2ArrayOfSignals7/1(ArrayofElements) -> Spare_3/1
  Bus Selector/8 -> Signal2ArrayOfSignals8/2(Element)  "<Spare4>"
  Signal2ArrayOfSignals8/1(ArrayofElements) -> Spare_4/1
  Bus Selector/9 -> Signal2ArrayOfSignals9/2(Element)  "<Spare5>"
  Bus Selector/10 -> Signal2ArrayOfSignals10/2(Element)  "<Spare6>"
  Bus Selector/11 -> Signal2ArrayOfSignals11/2(Element)  "<Spare7>"
  Bus Selector/12 -> Signal2ArrayOfSignals12/2(Element)  "<Spare8>"
  Signal2ArrayOfSignals9/1(ArrayofElements) -> Spare_5/1
  Signal2ArrayOfSignals10/1(ArrayofElements) -> Spare_6/1
  Signal2ArrayOfSignals11/1(ArrayofElements) -> Spare_7/1
  Signal2ArrayOfSignals12/1(ArrayofElements) -> Spare_8/1
  Bus Selector/13 -> Signal2ArrayOfSignals13/2(Element)  "<Spare9>"
  Bus Selector/14 -> Signal2ArrayOfSignals14/2(Element)  "<Spare10>"
  Signal2ArrayOfSignals13/1(ArrayofElements) -> Spare_9/1
  Signal2ArrayOfSignals14/1(ArrayofElements) -> Spare_10/1
  Bus Selector/15 -> Signal2ArrayOfSignals15/2(Element)  "<Spare11>"
  Signal2ArrayOfSignals15/1(ArrayofElements) -> Spare_11/1
  Bus Selector/16 -> Signal2ArrayOfSignals16/2(Element)  "<Spare12>"
  Signal2ArrayOfSignals16/1(ArrayofElements) -> Spare_12/1
  Bus Selector/17 -> Signal2ArrayOfSignals17/2(Element)  "<Spare13>"
  Signal2ArrayOfSignals17/1(ArrayofElements) -> Spare_13/1
  Bus Selector/18 -> Signal2ArrayOfSignals18/2(Element)  "<Spare14>"
  Signal2ArrayOfSignals18/1(ArrayofElements) -> Spare_14/1
  Bus Selector/19 -> Signal2ArrayOfSignals19/2(Element)  "<Spare15>"
  Signal2ArrayOfSignals19/1(ArrayofElements) -> Spare_15/1

== system Demo_TollSystem_cs/HighwayOverhang_3/RFBeacon_3_Tx_Mux ==
  BeaconType : Inport
  Spare_1 : Inport  Port=2
  Spare_2 : Inport  Port=3
  Spare_3 : Inport  Port=4
  Spare_4 : Inport  Port=5
  Spare_5 : Inport  Port=6
  Spare_6 : Inport  Port=7
  Spare_7 : Inport  Port=8
  Spare_8 : Inport  Port=9
  Spare_9 : Inport  Port=10
  Spare_10 : Inport  Port=11
  Spare_11 : Inport  Port=12
  Spare_12 : Inport  Port=13
  Spare_13 : Inport  Port=14
  Spare_14 : Inport  Port=15
  Spare_15 : Inport  Port=16
  Bus Creator : BusCreator  Inputs=16  OutDataTypeStr=Bus: PRESCAN_BEACONOBU_INPUT_DATA
  BeaconTx : Outport
  wires:
  Spare_11/1 -> Bus Creator/12  "Spare11"
  Spare_12/1 -> Bus Creator/13  "Spare12"
  Spare_13/1 -> Bus Creator/14  "Spare13"
  Spare_14/1 -> Bus Creator/15  "Spare14"
  Spare_15/1 -> Bus Creator/16  "Spare15"
  Spare_1/1 -> Bus Creator/2  "Spare1"
  Spare_2/1 -> Bus Creator/3  "Spare2"
  Spare_3/1 -> Bus Creator/4  "Spare3"
  Spare_4/1 -> Bus Creator/5  "Spare4"
  Spare_5/1 -> Bus Creator/6  "Spare5"
  Spare_6/1 -> Bus Creator/7  "Spare6"
  Spare_7/1 -> Bus Creator/8  "Spare7"
  Spare_8/1 -> Bus Creator/9  "Spare8"
  Spare_9/1 -> Bus Creator/10  "Spare9"
  Spare_10/1 -> Bus Creator/11  "Spare10"
  Bus Creator/1 -> BeaconTx/1
  BeaconType/1 -> Bus Creator/1  "TypeID"

== system Demo_TollSystem_cs/HighwayOverhang_3/threshold check ==
  Lat : Inport
  Lon : Inport  Port=2
  Pos Lat : Inport  Port=3
  Pos Lon : Inport  Port=4
  Abs : Abs
  Abs1 : Abs
  Accuracy : Constant  Value=1e-5
  Compare To Zero : simulink/Logic and Bit Operations/Compare To Zero  relop=~=  OutDataTypeStr=uint8  ZeroCross=off
  Compare To Zero1 : simulink/Logic and Bit Operations/Compare To Zero  relop=~=  OutDataTypeStr=uint8  ZeroCross=off
  Logical Operator : Logic  Inputs=3  AllPortsSameDT=off  OutDataTypeStr=float('double')
  Logical Operator1 : Logic  Operator=OR  AllPortsSameDT=off  OutDataTypeStr=boolean
  Relational Operator : RelationalOperator  Operator=>  OutDataTypeStr=boolean
  Relational Operator1 : RelationalOperator  Operator=>  OutDataTypeStr=boolean
  Sum : Sum  Inputs=|+-
  Sum1 : Sum  Inputs=|+-
  Out : Outport
  wires:
  Pos Lat/1 -> Sum/2
  Lat/1 -> Sum/1, Compare To Zero/1
  Sum/1 -> Abs/1
  Pos Lon/1 -> Sum1/2
  Lon/1 -> Sum1/1, Compare To Zero1/1
  Sum1/1 -> Abs1/1
  Relational Operator/1 -> Logical Operator1/1
  Logical Operator/1 -> Out/1
  Abs/1 -> Relational Operator/1
  Accuracy/1 -> Relational Operator/2, Relational Operator1/2
  Abs1/1 -> Relational Operator1/1
  Compare To Zero/1 -> Logical Operator/1
  Compare To Zero1/1 -> Logical Operator1/2
  Relational Operator1/1 -> Logical Operator/3
  Logical Operator1/1 -> Logical Operator/2

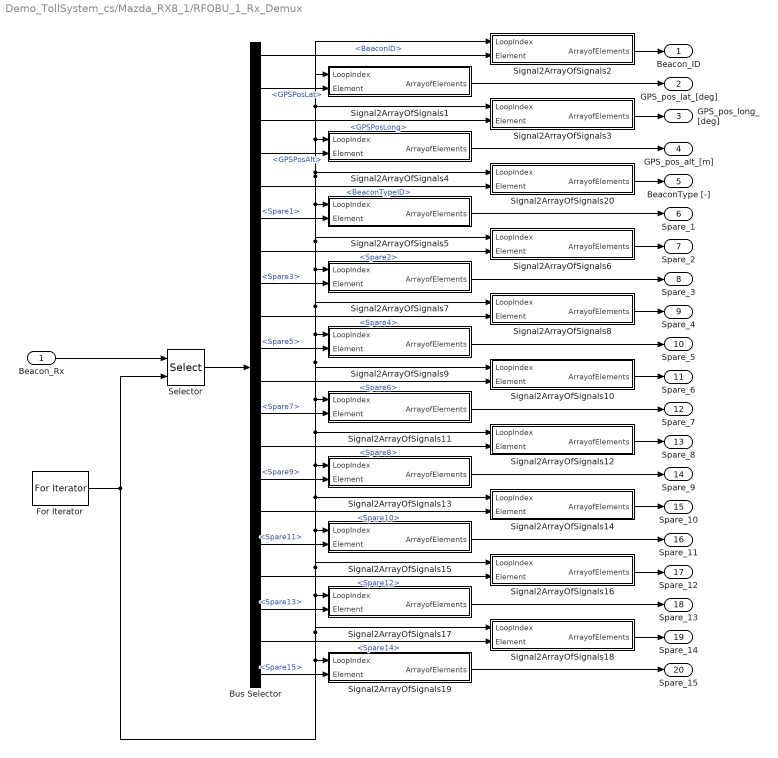
== system Demo_TollSystem_cs/Mazda_RX8_1/RFOBU_1_Rx_Demux ==
  Beacon_Rx : Inport
  Bus Selector : BusSelector  OutputSignals=DATA.BeaconID,DATA.GPSPosLat,DATA.GPSPosLong,DATA.GPSPosAlt,DATA.BeaconTypeID,DATA.Spare1,DATA.Spare2,DATA.Spare3,DATA.Spare4,DATA.Spare5,DATA.Spare6,DATA.Spare7,DATA.Spare8,DATA.Spare9,DATA.Spare10,DATA.Spare11,DATA.Spare12,DATA.Spare13,DATA.Spare14,DATA.Spare15
  For Iterator : ForIterator  ResetStates=reset  IterationLimit=detectableObjects
  Selector : Selector  InputPortWidth=detectableObjects  IndexOptions=Index vector (port)  Indices=[1 3]
  Signal2ArrayOfSignals1 : Subsystem  mask{VECTORLENGTH=detectableObjects}
      mask prompts: VECTORLENGTH "Length of vector"
  Signal2ArrayOfSignals10 : Subsystem  mask{VECTORLENGTH=detectableObjects}
      mask prompts: VECTORLENGTH "Length of vector"
  Signal2ArrayOfSignals11 : Subsystem  mask{VECTORLENGTH=detectableObjects}
      mask prompts: VECTORLENGTH "Length of vector"
  Signal2ArrayOfSignals12 : Subsystem  mask{VECTORLENGTH=detectableObjects}
      mask prompts: VECTORLENGTH "Length of vector"
  Signal2ArrayOfSignals13 : Subsystem  mask{VECTORLENGTH=detectableObjects}
      mask prompts: VECTORLENGTH "Length of vector"
  Signal2ArrayOfSignals14 : Subsystem  mask{VECTORLENGTH=detectableObjects}
      mask prompts: VECTORLENGTH "Length of vector"
  Signal2ArrayOfSignals15 : Subsystem  mask{VECTORLENGTH=detectableObjects}
      mask prompts: VECTORLENGTH "Length of vector"
  Signal2ArrayOfSignals16 : Subsystem  mask{VECTORLENGTH=detectableObjects}
      mask prompts: VECTORLENGTH "Length of vector"
  Signal2ArrayOfSignals17 : Subsystem  mask{VECTORLENGTH=detectableObjects}
      mask prompts: VECTORLENGTH "Length of vector"
  Signal2ArrayOfSignals18 : Subsystem  mask{VECTORLENGTH=detectableObjects}
      mask prompts: VECTORLENGTH "Length of vector"
  Signal2ArrayOfSignals19 : Subsystem  mask{VECTORLENGTH=detectableObjects}
      mask prompts: VECTORLENGTH "Length of vector"
  Signal2ArrayOfSignals2 : Subsystem  mask{VECTORLENGTH=detectableObjects}
      mask prompts: VECTORLENGTH "Length of vector"
  Signal2ArrayOfSignals20 : Subsystem  mask{VECTORLENGTH=detectableObjects}
      mask prompts: VECTORLENGTH "Length of vector"
  Signal2ArrayOfSignals3 : Subsystem  mask{VECTORLENGTH=detectableObjects}
      mask prompts: VECTORLENGTH "Length of vector"
  Signal2ArrayOfSignals4 : Subsystem  mask{VECTORLENGTH=detectableObjects}
      mask prompts: VECTORLENGTH "Length of vector"
  Signal2ArrayOfSignals5 : Subsystem  mask{VECTORLENGTH=detectableObjects}
      mask prompts: VECTORLENGTH "Length of vector"
  Signal2ArrayOfSignals6 : Subsystem  mask{VECTORLENGTH=detectableObjects}
      mask prompts: VECTORLENGTH "Length of vector"
  Signal2ArrayOfSignals7 : Subsystem  mask{VECTORLENGTH=detectableObjects}
      mask prompts: VECTORLENGTH "Length of vector"
  Signal2ArrayOfSignals8 : Subsystem  mask{VECTORLENGTH=detectableObjects}
      mask prompts: VECTORLENGTH "Length of vector"
  Signal2ArrayOfSignals9 : Subsystem  mask{VECTORLENGTH=detectableObjects}
      mask prompts: VECTORLENGTH "Length of vector"
  Beacon_ID : Outport
  GPS_pos_lat_[deg] : Outport  Port=2
  GPS_pos_long_[deg] : Outport  Port=3
  GPS_pos_alt_[m] : Outport  Port=4
  BeaconType [-] : Outport  Port=5
  Spare_1 : Outport  Port=6
  Spare_2 : Outport  Port=7
  Spare_3 : Outport  Port=8
  Spare_4 : Outport  Port=9
  Spare_5 : Outport  Port=10
  Spare_6 : Outport  Port=11
  Spare_7 : Outport  Port=12
  Spare_8 : Outport  Port=13
  Spare_9 : Outport  Port=14
  Spare_10 : Outport  Port=15
  Spare_11 : Outport  Port=16
  Spare_12 : Outport  Port=17
  Spare_13 : Outport  Port=18
  Spare_14 : Outport  Port=19
  Spare_15 : Outport  Port=20
  wires:
  Beacon_Rx/1 -> Selector/1
  For Iterator/1 -> Selector/2, Signal2ArrayOfSignals19/1(LoopIndex), Signal2ArrayOfSignals17/1(LoopIndex), Signal2ArrayOfSignals15/1(LoopIndex), Signal2ArrayOfSignals13/1(LoopIndex), Signal2ArrayOfSignals11/1(LoopIndex), Signal2ArrayOfSignals9/1(LoopIndex), Signal2ArrayOfSignals7/1(LoopIndex), Signal2ArrayOfSignals5/1(LoopIndex), Signal2ArrayOfSignals4/1(LoopIndex), Signal2ArrayOfSignals3/1(LoopIndex), Signal2ArrayOfSignals2/1(LoopIndex), Signal2ArrayOfSignals1/1(LoopIndex), Signal2ArrayOfSignals20/1(LoopIndex), Signal2ArrayOfSignals6/1(LoopIndex), Signal2ArrayOfSignals8/1(LoopIndex), Signal2ArrayOfSignals10/1(LoopIndex), Signal2ArrayOfSignals12/1(LoopIndex), Signal2ArrayOfSignals14/1(LoopIndex), Signal2ArrayOfSignals16/1(LoopIndex), Signal2ArrayOfSignals18/1(LoopIndex)
  Selector/1 -> Bus Selector/1
  Bus Selector/1 -> Signal2ArrayOfSignals2/2(Element)  "<BeaconID>"
  Signal2ArrayOfSignals2/1(ArrayofElements) -> Beacon_ID/1
  Bus Selector/2 -> Signal2ArrayOfSignals1/2(Element)  "<GPSPosLat>"
  Signal2ArrayOfSignals1/1(ArrayofElements) -> GPS_pos_lat_[deg]/1
  Bus Selector/3 -> Signal2ArrayOfSignals3/2(Element)  "<GPSPosLong>"
  Signal2ArrayOfSignals3/1(ArrayofElements) -> GPS_pos_long_[deg]/1
  Bus Selector/4 -> Signal2ArrayOfSignals4/2(Element)  "<GPSPosAlt>"
  Signal2ArrayOfSignals4/1(ArrayofElements) -> GPS_pos_alt_[m]/1
  Bus Selector/6 -> Signal2ArrayOfSignals5/2(Element)  "<Spare1>"
  Signal2ArrayOfSignals5/1(ArrayofElements) -> Spare_1/1
  Bus Selector/7 -> Signal2ArrayOfSignals6/2(Element)  "<Spare2>"
  Signal2ArrayOfSignals6/1(ArrayofElements) -> Spare_2/1
  Bus Selector/8 -> Signal2ArrayOfSignals7/2(Element)  "<Spare3>"
  Signal2ArrayOfSignals7/1(ArrayofElements) -> Spare_3/1
  Bus Selector/9 -> Signal2ArrayOfSignals8/2(Element)  "<Spare4>"
  Signal2ArrayOfSignals8/1(ArrayofElements) -> Spare_4/1
  Bus Selector/10 -> Signal2ArrayOfSignals9/2(Element)  "<Spare5>"
  Bus Selector/11 -> Signal2ArrayOfSignals10/2(Element)  "<Spare6>"
  Bus Selector/12 -> Signal2ArrayOfSignals11/2(Element)  "<Spare7>"
  Bus Selector/13 -> Signal2ArrayOfSignals12/2(Element)  "<Spare8>"
  Signal2ArrayOfSignals9/1(ArrayofElements) -> Spare_5/1
  Signal2ArrayOfSignals10/1(ArrayofElements) -> Spare_6/1
  Signal2ArrayOfSignals11/1(ArrayofElements) -> Spare_7/1
  Signal2ArrayOfSignals12/1(ArrayofElements) -> Spare_8/1
  Bus Selector/14 -> Signal2ArrayOfSignals13/2(Element)  "<Spare9>"
  Bus Selector/15 -> Signal2ArrayOfSignals14/2(Element)  "<Spare10>"
  Signal2ArrayOfSignals13/1(ArrayofElements) -> Spare_9/1
  Signal2ArrayOfSignals14/1(ArrayofElements) -> Spare_10/1
  Bus Selector/16 -> Signal2ArrayOfSignals15/2(Element)  "<Spare11>"
  Signal2ArrayOfSignals15/1(ArrayofElements) -> Spare_11/1
  Bus Selector/17 -> Signal2ArrayOfSignals16/2(Element)  "<Spare12>"
  Signal2ArrayOfSignals16/1(ArrayofElements) -> Spare_12/1
  Bus Selector/18 -> Signal2ArrayOfSignals17/2(Element)  "<Spare13>"
  Signal2ArrayOfSignals17/1(ArrayofElements) -> Spare_13/1
  Bus Selector/19 -> Signal2ArrayOfSignals18/2(Element)  "<Spare14>"
  Signal2ArrayOfSignals18/1(ArrayofElements) -> Spare_14/1
  Bus Selector/20 -> Signal2ArrayOfSignals19/2(Element)  "<Spare15>"
  Signal2ArrayOfSignals19/1(ArrayofElements) -> Spare_15/1
  Bus Selector/5 -> Signal2ArrayOfSignals20/2(Element)  "<BeaconTypeID>"
  Signal2ArrayOfSignals20/1(ArrayofElements) -> BeaconType [-]/1

== system Demo_TollSystem_cs/Mazda_RX8_1/RFOBU_1_Tx_Mux ==
  Vehicle_Type : Inport
  Spare_1 : Inport  Port=2
  Spare_2 : Inport  Port=3
  Spare_3 : Inport  Port=4
  Spare_4 : Inport  Port=5
  Spare_5 : Inport  Port=6
  Spare_6 : Inport  Port=7
  Spare_7 : Inport  Port=8
  Spare_8 : Inport  Port=9
  Spare_9 : Inport  Port=10
  Spare_10 : Inport  Port=11
  Spare_11 : Inport  Port=12
  Spare_12 : Inport  Port=13
  Spare_13 : Inport  Port=14
  Spare_14 : Inport  Port=15
  Spare_15 : Inport  Port=16
  Bus Creator : BusCreator  Inputs=16  OutDataTypeStr=Bus: PRESCAN_BEACONOBU_INPUT_DATA
  BeaconTx : Outport
  wires:
  Vehicle_Type/1 -> Bus Creator/1  "TypeID"
  Bus Creator/1 -> BeaconTx/1
  Spare_10/1 -> Bus Creator/11  "Spare10"
  Spare_9/1 -> Bus Creator/10  "Spare9"
  Spare_8/1 -> Bus Creator/9  "Spare8"
  Spare_7/1 -> Bus Creator/8  "Spare7"
  Spare_6/1 -> Bus Creator/7  "Spare6"
  Spare_5/1 -> Bus Creator/6  "Spare5"
  Spare_4/1 -> Bus Creator/5  "Spare4"
  Spare_3/1 -> Bus Creator/4  "Spare3"
  Spare_2/1 -> Bus Creator/3  "Spare2"
  Spare_1/1 -> Bus Creator/2  "Spare1"
  Spare_15/1 -> Bus Creator/16  "Spare15"
  Spare_14/1 -> Bus Creator/15  "Spare14"
  Spare_13/1 -> Bus Creator/14  "Spare13"
  Spare_12/1 -> Bus Creator/13  "Spare12"
  Spare_11/1 -> Bus Creator/12  "Spare11"

== system Demo_TollSystem_cs/Mazda_RX8_1/S-Memory ==
  note: Memory:
      | - If Set >0 or Rising (switchable)
      |     Out = Signal
      | - Else
      |     Out = Previous Signal
      | - End
  Set : Inport
  Signal : Inport  Port=2
  Detect Rise Positive : simulink/Logic and Bit Operations/Detect Rise Positive  vinit=0  InputProcessing=Inherited  OutDataTypeStr=uint8
  Manual Switch : ManualSwitch
  Switch : Switch  Criteria=u2 ~= 0
  Unit Delay : UnitDelay  SampleTime=-1
  Out : Outport
  wires:
  Manual Switch/1 -> Switch/2
  Detect Rise Positive/1 -> Manual Switch/1
  Set/1 -> Manual Switch/2, Detect Rise Positive/1
  Unit Delay/1 -> Switch/3
  Signal/1 -> Switch/1
  Switch/1 -> Unit Delay/1, Out/1

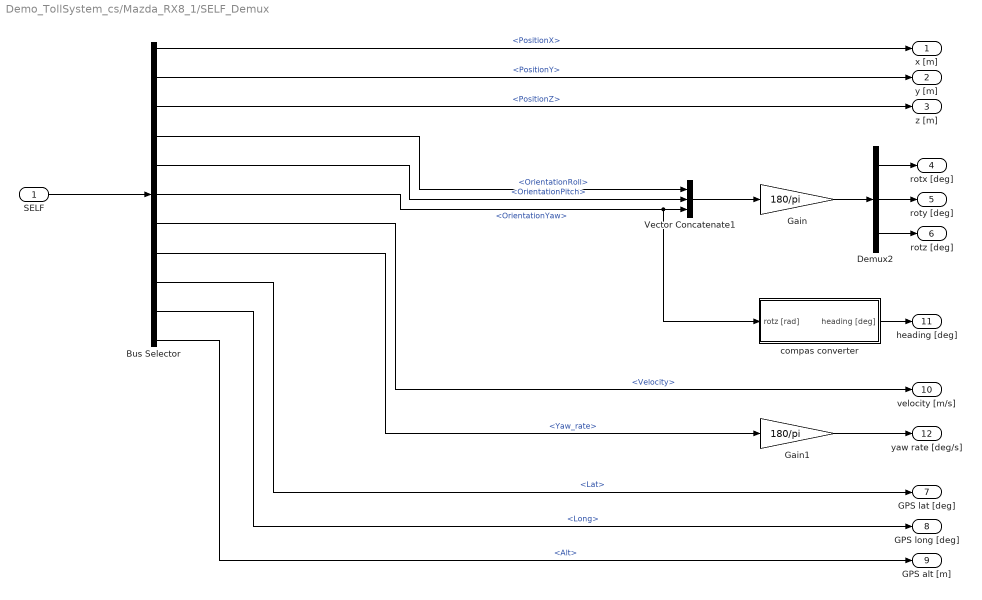
== system Demo_TollSystem_cs/Mazda_RX8_1/SELF_Demux ==
  SELF : Inport  OutDataTypeStr=Bus: PRESCAN_SELFSENSORDATA
  Bus Selector : BusSelector  OutputSignals=PositionX,PositionY,PositionZ,OrientationRoll,OrientationPitch,OrientationYaw,Velocity,Yaw_rate,Lat,Long,Alt
  Demux2 : Demux  Outputs=3
  Gain : Gain  Gain=180/pi
  Gain1 : Gain  Gain=180/pi
  Vector Concatenate1 : Concatenate  NumInputs=3
  compas converter : Subsystem
  x [m] : Outport
  y [m] : Outport  Port=2
  z [m] : Outport  Port=3
  rotx [deg] : Outport  Port=4
  roty [deg] : Outport  Port=5
  rotz [deg] : Outport  Port=6
  GPS lat [deg] : Outport  Port=7
  GPS long [deg] : Outport  Port=8
  GPS alt [m] : Outport  Port=9
  velocity [m/s] : Outport  Port=10
  heading [deg] : Outport  Port=11
  yaw rate [deg/s] : Outport  Port=12
  wires:
  Bus Selector/11 -> GPS alt [m]/1  "<Alt>"
  Bus Selector/10 -> GPS long [deg]/1  "<Long>"
  Bus Selector/9 -> GPS lat [deg]/1  "<Lat>"
  Bus Selector/8 -> Gain1/1  "<Yaw_rate>"
  Bus Selector/7 -> velocity [m/s]/1  "<Velocity>"
  Bus Selector/6 -> compas converter/1(rotz [rad]), Vector Concatenate1/3  "<OrientationYaw>"
  Bus Selector/5 -> Vector Concatenate1/2  "<OrientationPitch>"
  Bus Selector/4 -> Vector Concatenate1/1  "<OrientationRoll>"
  Vector Concatenate1/1 -> Gain/1
  Bus Selector/3 -> z [m]/1  "<PositionZ>"
  Bus Selector/2 -> y [m]/1  "<PositionY>"
  Bus Selector/1 -> x [m]/1  "<PositionX>"
  SELF/1 -> Bus Selector/1
  Gain/1 -> Demux2/1
  Demux2/1 -> rotx [deg]/1
  Demux2/2 -> roty [deg]/1
  Demux2/3 -> rotz [deg]/1
  compas converter/1(heading [deg]) -> heading [deg]/1
  Gain1/1 -> yaw rate [deg/s]/1

== system Demo_TollSystem_cs/HighwayOverhang_1/RFBeacon_1_Rx_Demux/Signal2ArrayOfSignals1 ==
  note: Set mask parameter VECTORLENGTH
      |  to MAXMESSAGES
  note: Initial state of Previous vector block
      | set to zeros(VECTORLENGTH,1)
  LoopIndex : Inport
  Element : Inport  Port=2
  Assignment : Assignment  IndexOptions=Index vector (port)
  Previous vector : Memory  X0=zeros(VECTORLENGTH,1)  InheritSampleTime=on
  ArrayofElements : Outport
  wires:
  Element/1 -> Assignment/2
  LoopIndex/1 -> Assignment/3
  Previous vector/1 -> Assignment/1
  Assignment/1 -> ArrayofElements/1, Previous vector/1

== system Demo_TollSystem_cs/HighwayOverhang_1/RFBeacon_1_Rx_Demux/Signal2ArrayOfSignals10 ==
  note: Set mask parameter VECTORLENGTH
      |  to MAXMESSAGES
  note: Initial state of Previous vector block
      | set to zeros(VECTORLENGTH,1)
  LoopIndex : Inport
  Element : Inport  Port=2
  Assignment : Assignment  IndexOptions=Index vector (port)
  Previous vector : Memory  X0=zeros(VECTORLENGTH,1)  InheritSampleTime=on
  ArrayofElements : Outport
  wires:
  Element/1 -> Assignment/2
  LoopIndex/1 -> Assignment/3
  Previous vector/1 -> Assignment/1
  Assignment/1 -> ArrayofElements/1, Previous vector/1

== system Demo_TollSystem_cs/HighwayOverhang_1/RFBeacon_1_Rx_Demux/Signal2ArrayOfSignals11 ==
  note: Set mask parameter VECTORLENGTH
      |  to MAXMESSAGES
  note: Initial state of Previous vector block
      | set to zeros(VECTORLENGTH,1)
  LoopIndex : Inport
  Element : Inport  Port=2
  Assignment : Assignment  IndexOptions=Index vector (port)
  Previous vector : Memory  X0=zeros(VECTORLENGTH,1)  InheritSampleTime=on
  ArrayofElements : Outport
  wires:
  Element/1 -> Assignment/2
  LoopIndex/1 -> Assignment/3
  Previous vector/1 -> Assignment/1
  Assignment/1 -> ArrayofElements/1, Previous vector/1

== system Demo_TollSystem_cs/HighwayOverhang_1/RFBeacon_1_Rx_Demux/Signal2ArrayOfSignals12 ==
  note: Set mask parameter VECTORLENGTH
      |  to MAXMESSAGES
  note: Initial state of Previous vector block
      | set to zeros(VECTORLENGTH,1)
  LoopIndex : Inport
  Element : Inport  Port=2
  Assignment : Assignment  IndexOptions=Index vector (port)
  Previous vector : Memory  X0=zeros(VECTORLENGTH,1)  InheritSampleTime=on
  ArrayofElements : Outport
  wires:
  Element/1 -> Assignment/2
  LoopIndex/1 -> Assignment/3
  Previous vector/1 -> Assignment/1
  Assignment/1 -> ArrayofElements/1, Previous vector/1
